simulink model "Test_LED_Amine"  (R2020b)
settings: Solver=FixedStepDiscrete  StartTime=0.0  StopTime=10.0  FixedStep=0.00001  RelTol=1e-3
model workspace (MAT data in the model file):
  Imax = 1.5
  Vmax = 90
  Vout = 300
values from neighbouring files (symbols this model uses):
  V1_gain = Coef1(2)    [ADC_calibrate.m]
  V1_offset = Coef1(1)    [ADC_calibrate.m]
libraries: GPIO_Lib x2, HRTIMERS_Lib x1, ADC_Lib x1, DAC_Lib x1, STM32_Config_Lib x1, TIMERS_Lib x1
settings Model: Creator=fenard1  LastModifiedBy=jlabaisse
settings DataIOCC: ReturnWorkspaceOutputs=off
settings OptimizationCC: DefaultParameterBehavior=Inlined  DefaultUnderspecifiedDataType=single  EnhancedBackFolding=on  CachingGlobalReferences=on  PassReuseOutputArgsAs=Individual arguments  EfficientTunableParamExpr=on
settings DebuggingCC: MultiTaskDSMMsg=none  ParameterTunabilityLossMsg=error  UnnecessaryDatatypeConvMsg=warning  SFcnCompatibilityMsg=warning  UniqueDataStoreMsg=error  StrictBusMsg=ErrorOnBusTreatedAsVector  SFUndirectedBroadcastEventsDiag=error  ArithmeticOperatorsInVariantConditions=warning
settings HardwareCC: ProdBitPerPointer=32  ProdBitPerSizeT=32  ProdBitPerPtrDiffT=32  ProdLargestAtomicFloat=None  ProdWordSize=32  ProdHWDeviceType=Custom Processor->Custom Processor
settings ModelReferenceCC: PropagateSignalLabelsOutOfModel=off
settings SFSimCC: CompileTimeRecursionLimit=0  EnableRuntimeRecursion=off  MATLABDynamicMemAlloc=off  CustomCodeUndefinedFunction=UseInterfaceOnly
settings RTWCC: Description=stm32 (Embedded Target)  SystemTargetFile=stm32.tlc  TemplateMakefile=stm32.tmf  GenerateReport=on  IncludeHyperlinkInReport=on  GenerateTraceInfo=on  GenerateTraceReport=on  GenerateTraceReportSl=on  GenerateTraceReportSf=on  GenerateTraceReportEml=on
settings CodeAppCC: ForceParamTrailComments=on  IgnoreCustomStorageClasses=off  IgnoreTestpoints=on  OperatorAnnotations=on  SimulinkDataObjDesc=on  SFDataObjDesc=on  CustomSymbolStrType=$N$R$M  InsertBlockDesc=on
settings STFCustomTargetCC: TargetLangStandard=C99 (ISO)  CodeReplacementLibrary=ARM CMSIS SIN COS  MultiwordLength=256  ParMdlRefBuildCompliant=on  ConcurrentExecutionCompliant=off  IncludeMdlTerminateFcn=off  CombineOutputUpdateFcns=on  ERTCustomFileBanners=on  SupportComplex=off  SupportContinuousTime=off  SupportNonInlinedSFcns=off  RemoveDisableFunc=on  RemoveResetFunc=on  ParenthesesLevel=Maximum  CastingMode=Standards  MATLABClassNameForMDSCustomization=Simulink.SoftwareTarget.ERTCustomization  CPPClassGenCompliant=off  GRTInterface=off  SystemTargetFile=stm32.tlc
settings ERTTargetCC: TargetLangStandard=C99 (ISO)  CodeReplacementLibrary=ARM CMSIS SIN COS  CompOptLevelCompliant=off  ConcurrentExecutionCompliant=off  IncludeMdlTerminateFcn=off  SupportComplex=off  RemoveDisableFunc=on  ParenthesesLevel=Maximum  CastingMode=Standards  ModelStepFunctionPrototypeControlCompliant=off  CPPClassGenCompliant=off  UseToolchainInfoCompliant=off  ExtModeStaticAllocSize=256  ExtModeMexArgs=0,1,115200,10  InlinedParameterPlacement=NonHierarchical  ERTSrcFileBannerTemplate=sourceFileTemplate.cgt  ERTHdrFileBannerTemplate=sourceFileTemplate.cgt  ERTDataSrcFileTemplate=sourceFileTemplate.cgt  ERTDataHdrFileTemplate=sourceFileTemplate.cgt  ERTCustomFileTemplate=customRoutineProcess.tlc  PreserveExpressionOrder=on  EnableSignedRightShifts=off

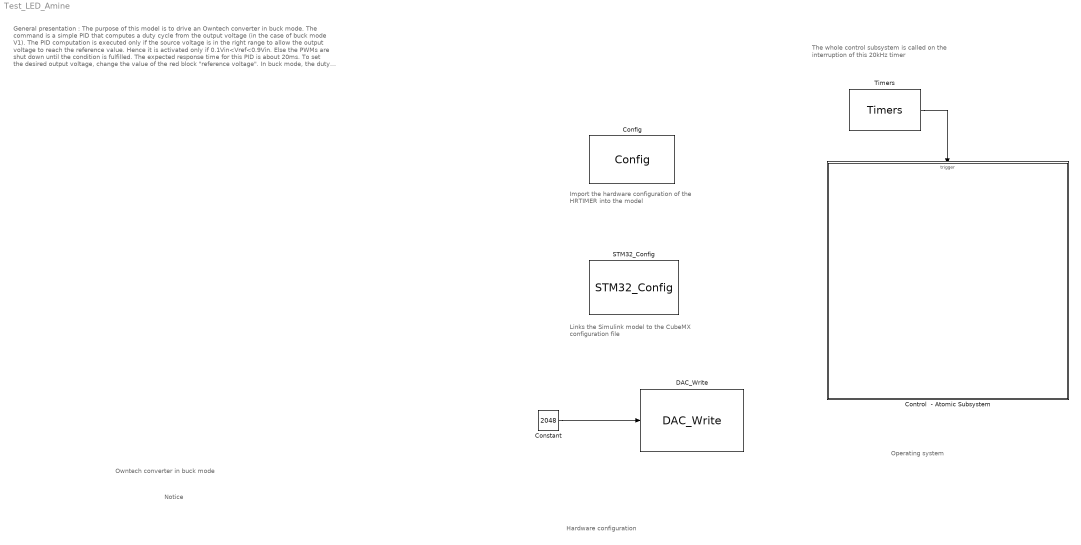
== system Test_LED_Amine ==
  note: Owntech converter in buck mode
  note: Notice
  note: Hardware configuration
  note: Operating system
  note: General presentation :
      |
      | The purpose of this model is to drive an Owntech converter in buck mode. The command is a simple PID that computes a duty cycle from the output voltage (in the case of buck mode V1). The PID computation is executed only if the source voltage is in the right range to allow the output voltage to reach the reference value. Hence it is activated only if 0.1Vin<Vref<0.9Vin. Else the PWMs are shut down until the condition is fulfilled.
      |
      | The expected response time for this PID is about 20ms.
      |
      | To set the desired output voltage, change the value of the red block "reference voltage".
      |
      | In buck mode, the duty cycle (corresponding to the PID_out) is the fraction of the period during which the high switches are ON (cf TI_Low1_H and TI_Low2_H on the scheme).
  note: Links the Simulink model to the CubeMX configuration file
  note: The whole control subsystem is called on the interruption of this 20kHz timer
  note: Import the hardware configuration of the HRTIMER into the model
  Config : HRTIMERS_Lib/Config  Priority=3  currentHRTIM=HRTIM1  NbHRTim=1  HRTIM_Name=HRTIM1  HRTIM_Clock=170000000  TIM_IRQ_F1=off  TIM_IRQ_F2=off  TIM_IRQ_F3=off  TIM_IRQ_F4=off  TIM_IRQ_F5=off  TIM_IRQ_F6=off  TIM_IRQ_SF=off  TIM_IRQ_BMP=off  TIM_IRQ_DLLCALL=off  TIM_IRQ_SYNC=off  TIM_IRQ_BURST_DMA=off  TIM_IRQ_DMA_ERR=off  M_DMA=off  M_IT_global=off  M_Tim_div=MUL16  M_Period=13600  M_PWM_Period=200000  M_Unit1=1360  M_Unit2=6800  M_Unit3=3000  M_Unit4=0  TIM_IRQ_UPDM=off  TIM_IRQ_REPM=off  TIM_IRQ_COMP1=off  TIM_IRQ_COMP2=off  TIM_IRQ_COMP3=off  TIM_IRQ_COMP4=off  A_Mode=Advanced  A_DMA=off  A_IT_global=off  A_Tim_div=MUL16  A_Period=13600  A_PWM_Period=200000  A_Capture1=off  A_Capture2=off  TA1_Enable=on  TA1_Polarity=HIGH  TA1_Chopper=off  TA2_Enable=on  TA2_Polarity=HIGH  TA2_Chopper=off  A_Unit1=6800  A_Unit2=0  A_Unit3=0  A_Unit4=0  A_Output_Comp1=off  A_Comp_Polarity1=HIGH  A_CompVal1=0  A_Output_Comp2=off  A_Comp_Polarity2=HIGH  A_CompVal2=0  A_Output_PWM1=off  A_Output_Polarity1=HIGH  A_DutyVal1=0  A_DutyIn1=off  A_Output_PWM2=off  A_Output_Polarity2=HIGH  A_DutyVal2=0  A_DutyIn2=off  A_OnePulse1=off  A_OnePulse_Polarity1=HIGH  A_OnePulse_CompVal1=0  A_OnePulse2=off  A_OnePulse_Polarity2=HIGH  A_OnePulse_CompVal2=0  TIM_IRQ_UPDA=off  TIM_IRQ_REPA=off  TIM_IRQ_COMP1A=off  TIM_IRQ_COMP2A=off  TIM_IRQ_COMP3A=off  TIM_IRQ_COMP4A=off  TIM_IRQ_CAPT1A=off  TIM_IRQ_CAPT2A=off  TIM_IRQ_DELA=off  TIM_IRQ_RESET_CPTA=off  TIM_IRQ_OUT1SA=off  TIM_IRQ_OUT1RA=off  TIM_IRQ_OUT2SA=off  TIM_IRQ_OUT2RA=off  B_Mode=Advanced  B_DMA=off  B_IT_global=off  B_Tim_div=MUL16  B_Period=13600  B_PWM_Period=200000  B_Capture1=off  B_Capture2=off  TB1_Enable=on  TB1_Polarity=HIGH  TB1_Chopper=off  TB2_Enable=on  TB2_Polarity=HIGH  TB2_Chopper=off  B_Unit1=6800  B_Unit2=0  B_Unit3=0  B_Unit4=0  B_Output_Comp1=off  B_Comp_Polarity1=HIGH  B_CompVal1=0  B_Output_Comp2=off  B_Comp_Polarity2=HIGH  B_CompVal2=0  B_Output_PWM1=off  B_Output_Polarity1=HIGH  B_DutyVal1=0  B_DutyIn1=off  B_Output_PWM2=off  B_Output_Polarity2=HIGH  B_DutyVal2=0  B_DutyIn2=off  B_OnePulse1=off  B_OnePulse_Polarity1=HIGH  B_OnePulse_CompVal1=0  B_OnePulse2=off  B_OnePulse_Polarity2=HIGH  B_OnePulse_CompVal2=0  TIM_IRQ_UPDB=off  TIM_IRQ_REPB=off  TIM_IRQ_COMP1B=off  TIM_IRQ_COMP2B=off  TIM_IRQ_COMP3B=off  TIM_IRQ_COMP4B=off  TIM_IRQ_CAPT1B=off  TIM_IRQ_CAPT2B=off  TIM_IRQ_DELB=off  TIM_IRQ_RESET_CPTB=off  TIM_IRQ_OUT1SB=off  TIM_IRQ_OUT1RB=off  TIM_IRQ_OUT2SB=off  TIM_IRQ_OUT2RB=off  C_Mode=Advanced  C_DMA=off  C_IT_global=off  C_Tim_div=MUL32  C_Period=0  C_PWM_Period=Inf  C_Capture1=off  C_Capture2=off  TC1_Enable=off  TC1_Polarity=HIGH  TC1_Chopper=off  TC2_Enable=off  TC2_Polarity=HIGH  TC2_Chopper=off  C_Unit1=0  C_Unit2=0  C_Unit3=0  C_Unit4=0  C_Output_Comp1=off  C_Comp_Polarity1=HIGH  C_CompVal1=0  C_Output_Comp2=off  C_Comp_Polarity2=HIGH  C_CompVal2=0  C_Output_PWM1=off  C_Output_Polarity1=HIGH  C_DutyVal1=0  C_DutyIn1=off  C_Output_PWM2=off  C_Output_Polarity2=HIGH  C_DutyVal2=0  C_DutyIn2=off  C_OnePulse1=off  C_OnePulse_Polarity1=HIGH  C_OnePulse_CompVal1=0  C_OnePulse2=off  C_OnePulse_Polarity2=HIGH  C_OnePulse_CompVal2=0  TIM_IRQ_UPDC=off  TIM_IRQ_REPC=off  TIM_IRQ_COMP1C=off  TIM_IRQ_COMP2C=off  TIM_IRQ_COMP3C=off  TIM_IRQ_COMP4C=off  TIM_IRQ_CAPT1C=off  TIM_IRQ_CAPT2C=off  TIM_IRQ_DELC=off  TIM_IRQ_RESET_CPTC=off  TIM_IRQ_OUT1SC=off  TIM_IRQ_OUT1RC=off  TIM_IRQ_OUT2SC=off  TIM_IRQ_OUT2RC=off  D_Mode=Advanced  D_DMA=off  D_IT_global=off  D_Tim_div=MUL32  D_Period=0  D_PWM_Period=Inf  D_Capture1=off  D_Capture2=off  TD1_Enable=off  TD1_Polarity=HIGH  TD1_Chopper=off  TD2_Enable=off  TD2_Polarity=HIGH  TD2_Chopper=off  D_Unit1=0  D_Unit2=0  D_Unit3=0  D_Unit4=0  D_Output_Comp1=off  D_Comp_Polarity1=HIGH  D_CompVal1=0  D_Output_Comp2=off  D_Comp_Polarity2=HIGH  D_CompVal2=0  D_Output_PWM1=off  D_Output_Polarity1=HIGH  D_DutyVal1=0  D_DutyIn1=off  D_Output_PWM2=off  D_Output_Polarity2=HIGH  D_DutyVal2=0  D_DutyIn2=off  D_OnePulse1=off  D_OnePulse_Polarity1=HIGH  D_OnePulse_CompVal1=0  D_OnePulse2=off  D_OnePulse_Polarity2=HIGH  D_OnePulse_CompVal2=0  TIM_IRQ_UPDD=off  TIM_IRQ_REPD=off  TIM_IRQ_COMP1D=off  TIM_IRQ_COMP2D=off  TIM_IRQ_COMP3D=off  TIM_IRQ_COMP4D=off  TIM_IRQ_CAPT1D=off  TIM_IRQ_CAPT2D=off  TIM_IRQ_DELD=off  TIM_IRQ_RESET_CPTD=off  TIM_IRQ_OUT1SD=off  TIM_IRQ_OUT1RD=off  TIM_IRQ_OUT2SD=off  TIM_IRQ_OUT2RD=off  E_Mode=Advanced  E_DMA=off  E_IT_global=off  E_Tim_div=MUL32  E_Period=0  E_PWM_Period=Inf  E_Capture1=off  E_Capture2=off  TE1_Enable=off  TE1_Polarity=HIGH  TE1_Chopper=off  TE2_Enable=off  TE2_Polarity=HIGH  TE2_Chopper=off  E_Unit1=0  E_Unit2=0  E_Unit3=0  E_Unit4=0  E_Output_Comp1=off  E_Comp_Polarity1=HIGH  E_CompVal1=0  E_Output_Comp2=off  E_Comp_Polarity2=HIGH  E_CompVal2=0  E_Output_PWM1=off  E_Output_Polarity1=HIGH  E_DutyVal1=0  E_DutyIn1=off  E_Output_PWM2=off  E_Output_Polarity2=HIGH  E_DutyVal2=0  E_DutyIn2=off  E_OnePulse1=off  E_OnePulse_Polarity1=HIGH  E_OnePulse_CompVal1=0  E_OnePulse2=off  E_OnePulse_Polarity2=HIGH  E_OnePulse_CompVal2=0  TIM_IRQ_UPDE=off  TIM_IRQ_REPE=off  TIM_IRQ_COMP1E=off  TIM_IRQ_COMP2E=off  TIM_IRQ_COMP3E=off  TIM_IRQ_COMP4E=off  TIM_IRQ_CAPT1E=off  TIM_IRQ_CAPT2E=off  TIM_IRQ_DELE=off  TIM_IRQ_RESET_CPTE=off  TIM_IRQ_OUT1SE=off  TIM_IRQ_OUT1RE=off  TIM_IRQ_OUT2SE=off  TIM_IRQ_OUT2RE=off  F_Mode=Advanced  F_DMA=off  F_IT_global=off  F_Tim_div=MUL32  F_Period=0  F_PWM_Period=Inf  F_Capture1=off  F_Capture2=off  TF1_Enable=off  TF1_Polarity=HIGH  TF1_Chopper=off  TF2_Enable=off  TF2_Polarity=HIGH  TF2_Chopper=off  F_Unit1=0  F_Unit2=0  F_Unit3=0  F_Unit4=0  F_Output_Comp1=off  F_Comp_Polarity1=HIGH  F_CompVal1=0  F_Output_Comp2=off  F_Comp_Polarity2=HIGH  F_CompVal2=0  F_Output_PWM1=off  F_Output_Polarity1=HIGH  F_DutyVal1=0  F_DutyIn1=off  F_Output_PWM2=off  F_Output_Polarity2=HIGH  F_DutyVal2=0  F_DutyIn2=off  F_OnePulse1=off  F_OnePulse_Polarity1=HIGH  F_OnePulse_CompVal1=0  F_OnePulse2=off  F_OnePulse_Polarity2=HIGH  F_OnePulse_CompVal2=0  TIM_IRQ_UPDF=off  TIM_IRQ_REPF=off  TIM_IRQ_COMP1F=off  TIM_IRQ_COMP2F=off  TIM_IRQ_COMP3F=off  TIM_IRQ_COMP4F=off  TIM_IRQ_CAPT1F=off  TIM_IRQ_CAPT2F=off  TIM_IRQ_DELF=off  TIM_IRQ_RESET_CPTF=off  TIM_IRQ_OUT1SF=off  TIM_IRQ_OUT1RF=off  TIM_IRQ_OUT2SF=off  TIM_IRQ_OUT2RF=off  M_Used=on  A_Used=on  B_Used=on  C_Used=off  D_Used=off  E_Used=off  F_Used=off
      settings: SourceProductName=Target Support Package - STM32 Adapter
  Constant : Constant  Value=2048  OutDataTypeStr=uint16
  Control  - Atomic Subsystem : Subsystem  Priority=1  TreatAsAtomicUnit=on  SystemSampleTime=1/50000
  DAC_Write : DAC_Lib/DAC_Write  DAC_Name=DAC2  Pin0=on  Pin1=off  Align=12bit_right  DmaBuffCh1=0  DmaBuffCh2=0  CpltTrans=off  HalfTrans=off  ErrorIt=off  UnderIt=off  NbDAC=1  UsedDma=off
      settings: SourceProductName=Target Support Package - STM32 Adapter
  STM32_Config : STM32_Config_Lib/STM32_Config  Priority=0  Project_Path=.\  Config_File=Test_LED_Amine.ioc  MCU_Name=STM32G474RETx
      settings: SourceProductName=Target Support Package - STM32 Adapter
  Timers : TIMERS_Lib/Timers  currentTIM=TIM3  TIM_Name=TIM3  sysUsingTimer=on  TIM_APBClock=170000000  TIM_Set_Clk=off  TIM_Prescaler=1023  TIM_Clock=166015.63  Variable_frequency=off  TIM_Set_OutFreq=on  TIM_ARR=166015  Output_frequency=1.00  Repetition_counter=0  TIM_Mode=Up  TIM_DMA=none  TIM_IRQ=on  TIM_IRQ_ONLY=off  TIM_UP=on  TIM_TRG=off  TIM_COM=off  TIM_BRK=off  NbTIM=1  CH1_enable=on  CH1N_enable=off  CH1_type=Output_PWM  CH1_DMA=off  CH1_int=off  CH1_edge=Rising  CH1_div=1  CH1_variable_duty=off  CH1_set_pulse=on  CH1_output_duty=50  CH1_pulse=83007  CH2_enable=off  CH2N_enable=off  CH2_type=Unknown  CH2_DMA=off  CH2_int=off  CH2_edge=Rising  CH2_div=1  CH2_variable_duty=off  CH2_set_pulse=off  CH2_output_duty=0.00  CH2_pulse=0  CH3_enable=off  CH3N_enable=off  CH3_type=Unknown  CH3_DMA=off  CH3_int=off  CH3_edge=Rising  CH3_div=1  CH3_variable_duty=off  CH3_set_pulse=off  CH3_output_duty=0.00  CH3_pulse=0  CH4_enable=off  CH4N_enable=off  CH4_type=Unknown  CH4_DMA=off  CH4_int=off  CH4_edge=Rising  CH4_div=1  CH4_variable_duty=off  CH4_set_pulse=off  CH4_output_duty=0.00  CH4_pulse=0
      settings: SourceProductName=Target Support Package - STM32 Adapter
  wires:
  Timers/1 -> Control  - Atomic Subsystem/Trigger
  Constant/1 -> DAC_Write/1

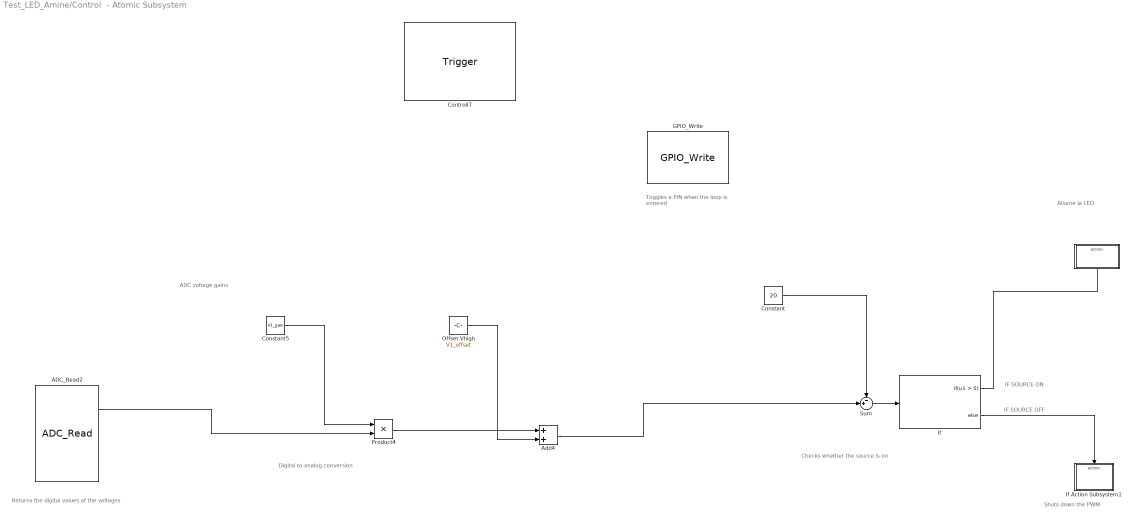
== system Test_LED_Amine/Control  - Atomic Subsystem ==
  note: IF SOURCE OFF
  note: IF SOURCE ON
  note: Checks whether the source is on
  note: Allume la LED
  note: Digital to analog conversion
  note: Shuts down the PWM
  note: Returns the digital values of the voltages
  note: ADC voltage gains
  note: Toggles a PIN when the loop is entered
  ControlIT : TriggerPort  TriggerType=function-call  VariantControl=Variant
  " " : Subsystem  TreatAsAtomicUnit=on
  ADC_Read2 : ADC_Lib/ADC_Read  ADC_Name=ADC2  ADC_Ch0=off  ADC_Ch1=on  ADC_Ch2=off  ADC_Ch3=off  ADC_Ch4=off  ADC_Ch5=off  ADC_Ch6=off  ADC_Ch7=off  ADC_Ch8=off  ADC_Ch9=off  ADC_Ch10=off  ADC_Ch11=off  ADC_Ch12=off  ADC_Ch13=off  ADC_Ch14=off  ADC_Ch15=off  ADC_Ch16=off  ADC_Ch17=off  ADC_Ch18=off  RgRk1=on  RgRk2=off  RgRk3=on  RgRk4=off  RgRk1_Ch=Ch1_r1  RgRk2_Ch=off  RgRk3_Ch=off  RgRk4_Ch=off  RgRk5=off  RgRk6=off  RgRk7=off  RgRk8=off  RgRk5_Ch=off  RgRk6_Ch=off  RgRk7_Ch=off  RgRk8_Ch=off  RgRk9=off  RgRk10=off  RgRk11=off  RgRk12=off  RgRk9_Ch=off  RgRk10_Ch=off  RgRk11_Ch=off  RgRk12_Ch=off  RgRk13=off  RgRk14=off  RgRk15=off  RgRk16=off  RgRk13_Ch=off  RgRk14_Ch=off  RgRk15_Ch=off  RgRk16_Ch=off  InjRk1=off  InjRk2=off  InjRk3=off  InjRk4=off  InjRk1_Ch=off  InjRk2_Ch=off  InjRk3_Ch=off  InjRk4_Ch=off  ADC_Trig=HRTIM_TRG1  ADC_TrigEdge=RISING  DmaReq=on  DMA_Buffer=3  ItReq=on  AWD_Mode=NOT_USED  AWD_Ch=0  AWD_HThres=0  AWD_LThres=0  AWD_En_Int=off  AWD2_HThres=0  AWD2_LThres=0  AWD2_En_Int=off  AWD3_HThres=0  AWD3_LThres=0  AWD3_En_Int=off  EOC_SEQ=off  EOC_IT=off  JEOC_IT=off  AWD_IT=off  OVR_IT=off  CpltTrans=off  HalfTrans=off  ADC_RegNb=1  ADC_RegCh0=off  ADC_RegCh1=on  ADC_RegCh2=off  ADC_RegCh3=off  ADC_RegCh4=off  ADC_RegCh5=off  ADC_RegCh6=off  ADC_RegCh7=off  ADC_RegCh8=off  ADC_RegCh9=off  ADC_RegCh10=off  ADC_RegCh11=off  ADC_RegCh12=off  ADC_RegCh13=off  ADC_RegCh14=off  ADC_RegCh15=off  ADC_RegCh16=off  ADC_RegCh17=off  ADC_RegCh18=off  ADC_InjNb=0  ADC_InjCh0=off  ADC_InjCh1=off  ADC_InjCh2=off  ADC_InjCh3=off  ADC_InjCh4=off  ADC_InjCh5=off  ADC_InjCh6=off  ADC_InjCh7=off  ADC_InjCh8=off  ADC_InjCh9=off  ADC_InjCh10=off  ADC_InjCh11=off  ADC_InjCh12=off  ADC_InjCh13=off  ADC_InjCh14=off  ADC_InjCh15=off  ADC_InjCh16=off  ADC_InjCh17=off  ADC_InjCh18=off  NbADC=1  CurrentADC=ADC2
      settings: SourceProductName=Target Support Package - STM32 Adapter
  Add4 : Sum  InputSameDT=on
  Constant : Constant  Value=20  OutDataTypeStr=single
  Constant5 : Constant  Value=V1_gain  OutDataTypeStr=single
  GPIO_Write : GPIO_Lib/GPIO_Write  Port_name=GPIOA  Pin0=off  Toggle_Pin0=off  Pin1=off  Toggle_Pin1=off  Pin2=off  Toggle_Pin2=off  Pin3=off  Toggle_Pin3=off  Pin4=off  Toggle_Pin4=off  Pin5=on  Toggle_Pin5=on  Pin6=off  Toggle_Pin6=off  Pin7=off  Toggle_Pin7=off  Pin8=off  Toggle_Pin8=off  Pin9=off  Toggle_Pin9=off  Pin10=off  Toggle_Pin10=off  Pin11=off  Toggle_Pin11=off  Pin12=off  Toggle_Pin12=off  Pin13=off  Toggle_Pin13=off  Pin14=off  Toggle_Pin14=off  Pin15=off  Toggle_Pin15=off  PinList=GPIOA5GPIOB11
      settings: SourceProductName=Target Support Package - STM32 Adapter
  If : If
  If Action Subsystem1 : Subsystem  TreatAsAtomicUnit=on
  Offset Vhigh : Constant  Value=V1_offset  OutDataTypeStr=single
  Product4 : Product  OutDataTypeStr=single
  Sum : Sum  Inputs=-+|  AccumDataTypeStr=single
  wires:
  Offset Vhigh/1 -> Add4/2
  Product4/1 -> Add4/1
  Constant5/1 -> Product4/1
  If/1 -> " "/Action
  If/2 -> If Action Subsystem1/Action
  Sum/1 -> If/1
  Add4/1 -> Sum/2
  Constant/1 -> Sum/1
  ADC_Read2/1 -> Product4/2

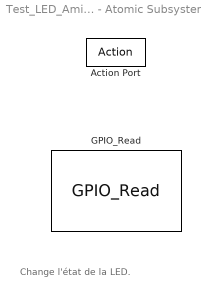
== system Test_LED_Amine/Control  - Atomic Subsystem/  ==
  note: Change l'état de la LED.
  Action Port : ActionPort  ActionPortLabel=if(u1 > 0)
  GPIO_Read : GPIO_Lib/GPIO_Read  Port_name=GPIOA  Pin_0=off  Pin_1=off  Pin_2=off  Pin_3=off  Pin_4=off  Pin_5=off  Pin_6=off  Pin_7=off  Pin_8=off  Pin_9=off  Pin_10=off  Pin_11=off  Pin_12=off  Pin_13=off  Pin_14=off  Pin_15=off  PinList=GPIOA0
      settings: SourceProductName=Target Support Package - STM32 Adapter

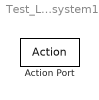
== system Test_LED_Amine/Control  - Atomic Subsystem/If Action Subsystem1 ==
  Action Port : ActionPort  ActionPortLabel=else
